simulink model "sldemo_pid2dof"  (R2019b)
settings: Solver=ode45  StartTime=0.0  StopTime=50  RelTol=1e-5  EnableMultiTasking=on
libraries: simulink x2
settings Model: Creator=The MathWorks, Inc.  LastModifiedBy=bhisma
settings DataIOCC: LimitDataPoints=on  MaxDataPoints=1100  SaveFormat=Array  ReturnWorkspaceOutputs=off
settings OptimizationCC: ExpressionDepthLimit=2147483647  LifeSpan=inf
settings DebuggingCC: FcnCallInpInsideContextMsg=warning  AllowSymbolicDim=off  StateNameClashWarn=warning  SFUnexpectedBacktrackingDiag=warning  SFNoUnconditionalDefaultTransitionDiag=warning  SFExecutionAtInitializationDiag=none  ArithmeticOperatorsInVariantConditions=warning
settings HardwareCC: ProdBitPerPointer=32  ProdBitPerSizeT=32  ProdBitPerPtrDiffT=32  ProdLargestAtomicFloat=None  ProdIntDivRoundTo=Undefined  ProdEndianess=Unspecified  ProdWordSize=32  ProdHWDeviceType=32-bit Generic
settings ModelReferenceCC: PropagateSignalLabelsOutOfModel=off
settings SFSimCC: SimUseLocalCustomCode=off  CustomCodeUndefinedFunction=UseInterfaceOnly
settings RTWCC: RTWUseLocalCustomCode=off
settings CodeAppCC: StateflowObjectComments=on
settings GRTTargetCC: TargetLangStandard=C89/C90 (ANSI)  GeneratePreprocessorConditionals=Disable all  CombineOutputUpdateFcns=off  GRTInterface=on
settings ConfigComp: CovMetricSettings=dw  CovHtmlReporting=on  CovSaveCumulativeToWorkspaceVar=on  CovSaveSingleToWorkspaceVar=on  CovExternalEMLEnable=off  CovSFcnEnable=off

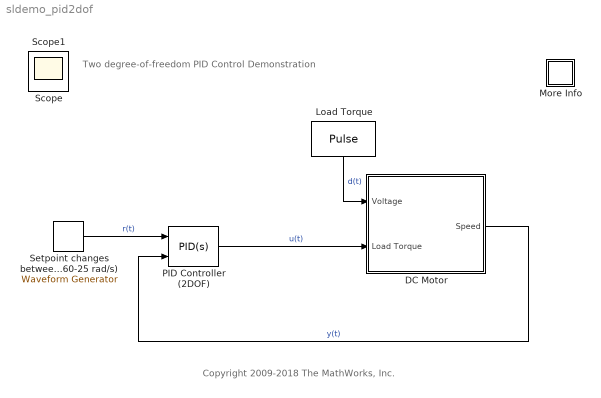
== system sldemo_pid2dof ==
  note: Two degree-of-freedom PID Control Demonstration
  note: Copyright 2009-2018 The MathWorks, Inc.
  DC Motor : Subsystem  mask(DC Motor){R=2, L=0.5, Km=0.1, Kf=0.2, J=0.02, Kb=0.1}
      mask prompts: R "R (Ohms)"; L "L (Henrys)"; Km "Km (Torque Constant)"; Kf "Kf (Nms)"; J "J (kg.m^2/s^2)"; Kb "Kb (Back emf Constant)"
      mask help: An ideal model of a DC Motor
      mask Help: This is <b>more elaborate<b> help.
      mask Display: image(fullfile(matlabroot,'toolbox','simulink','simdemos','industrial','images','maskIconDCMotor.png'))
  Load Torque : DiscretePulseGenerator  PulseType=Time based  Amplitude=-5  Period=10  PulseWidth=50  PhaseDelay=5
  More Info : Subsystem
      settings: OpenFcn=showdemo('sldemo_pid2dof')
      mask Display: disp('?')
  PID Controller (2DOF) : simulink/Continuous/PID Controller (2DOF)  Tag=PID1  Controller=PID  Form=Parallel  TimeDomain=Continuous-time  SampleTime=-1  IntegratorMethod=Forward Euler  FilterMethod=Forward Euler  ControllerParametersSource=internal  P=0.2  I=1.0  D=0.06  UseFilter=on  N=12  b=1  c=1  TunerSelectOption=Transfer Function Based (PID Tuner App)  ZeroCross=off  InitialConditionSource=internal  InitialConditionForIntegrator=0  InitialConditionForFilter=0  DifferentiatorICPrevScaledInput=0  ExternalReset=none  TrackingMode=off  Kt=1  LimitOutput=off  UpperSaturationLimit=inf  LowerSaturationLimit=-inf  LinearizeAsGain=off  AntiWindupMode=none  Kb=1  POutMin=[]  POutMax=[]  IOutMin=[]  IOutMax=[]  DOutMin=[]  DOutMax=[]  NOutMin=[]  NOutMax=[]  bOutMin=[]  bOutMax=[]  cOutMin=[]  cOutMax=[]  SumOutMin=[]  SumOutMax=[]  SaturationOutMin=[]  SaturationOutMax=[]  PParamMin=[]  PParamMax=[]  IParamMin=[]  IParamMax=[]  DParamMin=[]  DParamMax=[]  NParamMin=[]  NParamMax=[]  bParamMin=[]  bParamMax=[]  cParamMin=[]  cParamMax=[]  KbParamMin=[]  KbParamMax=[]  KtParamMin=[]  KtParamMax=[]  KbOutMin=[]  KbOutMax=[]  KtOutMin=[]  KtOutMax=[]  IntegratorOutMin=[]  IntegratorOutMax=[]  FilterOutMin=[]  FilterOutMax=[]  SumI1OutMin=[]  SumI1OutMax=[]  SumI2OutMin=[]  SumI2OutMax=[]  SumI3OutMin=[]  SumI3OutMax=[]  SumI4OutMin=[]  SumI4OutMax=[]  SumDOutMin=[]  SumDOutMax=[]  Sum1OutMin=[]  Sum1OutMax=[]  Sum2OutMin=[]  Sum2OutMax=[]  Sum3OutMin=[]  Sum3OutMax=[]  DifferentiatorOutMin=[]  DifferentiatorOutMax=[]  FilterDiffOutCoefMin=[]  FilterDiffOutCoefMax=[]  ReciprocalOutMin=[]  ReciprocalOutMax=[]  SumDenOutMin=[]  SumDenOutMax=[]  SumNumOutMin=[]  SumNumOutMax=[]  DivideOutMin=[]  DivideOutMax=[]  IntegratorContinuousStateAttributes=''  IntegratorStateMustResolveToSignalObject=off  IntegratorRTWStateStorageClass=Auto  FilterContinuousStateAttributes=''  FilterStateMustResolveToSignalObject=off  FilterRTWStateStorageClass=Auto  ParallelPVariant=InternalParameters  IdealPVariant=Disabled  IVariant=InternalParameters  DVariant=InternalParameters  bVariant=InternalParameters  cVariant=InternalParameters  IntegratorVariant=Continuous  SatVariant=Disabled  AWVariant=Passthrough  PCopyVariant=Disabled  TRVariant=Disabled  FdbkBlocksVariant=Forward  IdealPFdbkVariant=Disabled  SatFdbkVariant=Disabled  DerivativeFilterVariant=ContFilter  NVariant=InternalParameters  NCopyVariant=Disabled  FilterICVariant=InternalICsFilter  IntegratorICVariant=InternalICs  ExternalResetVariant=Disabled  TRSumVariant=Passthrough  SumFdbkVariant=Disabled  SumVariant=Sum_PID
  Setpoint changes between (60-25 rad/s) : simulink/Sources/Waveform Generator  OutMin=[]  OutMax=[]  OutDataTypeStr=double  SelectedSignal=1  Signals=step(10,60,25)+step(20,0,15)-step(30,0,10)  BlockNames=MultiportSwitch_88520505b6ef463  SampleTime=0.1
      settings: SourceProductName=Simulink
  Scope : Scope
  Scope1 : Scope
  wires:
  PID Controller (2DOF)/1 -> DC Motor/2(Load Torque)  "u(t)"
  Load Torque/1 -> DC Motor/1(Voltage)  "d(t)"
  Setpoint changes between (60-25 rad/s)/1 -> PID Controller (2DOF)/1  "r(t)"
  DC Motor/1(Speed) -> PID Controller (2DOF)/2  "y(t)"

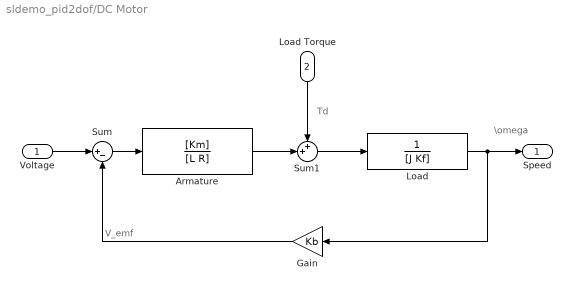
== system sldemo_pid2dof/DC Motor ==
  note: \omega
  note: V_emf
  note: Td
  Voltage : Inport
  Load Torque : Inport  Port=2
  Armature : TransferFcn  Numerator=[Km]  Denominator=[L R]
  Gain : Gain  Gain=Kb
  Load : TransferFcn  Denominator=[J Kf]
  Sum : Sum  Inputs=|+-
  Sum1 : Sum  Inputs=++|
  Speed : Outport  VectorParamsAs1DForOutWhenUnconnected=off
  wires:
  Load/1 -> Speed/1, Gain/1
  Load Torque/1 -> Sum1/1
  Armature/1 -> Sum1/2
  Sum1/1 -> Load/1
  Sum/1 -> Armature/1
  Voltage/1 -> Sum/1
  Gain/1 -> Sum/2

== system sldemo_pid2dof/More Info ==
